simulink model "computed_torque"  (Simulink 8.8)
settings: Solver=FixedStepDiscrete  StartTime=0.0  StopTime=inf  FixedStep=0.01  RelTol=1e-3
InitFcn:
  | WBT_modelName = 'computed-torque';
  | WBT_wbiList = 'ROBOT_TORQUE_CONTROL_JOINTS_WITHOUT_PRONOSUP';
  | 
  | setenv('YARP_ROBOT_NAME','icubGazeboSim');
  | 
  | Dofs = 23;
libraries: WBToolboxLibrary x3
settings Model: SuppressorTable=22 serialization::archive 11 0 3 0 0 0 0 0  Creator=makaveli  LastModifiedBy=makaveli
settings DataIOCC: LimitDataPoints=off  SaveFormat=Dataset  SignalLoggingSaveFormat=Dataset
settings OptimizationCC: LifeSpan=auto
settings DebuggingCC: UnderspecifiedInitializationDetection=Simplified  MergeDetectMultiDrivingBlocksExec=error  FcnCallInpInsideContextMsg=error  StateNameClashWarn=none  SFUnexpectedBacktrackingDiag=error  SFNoUnconditionalDefaultTransitionDiag=error  SFExecutionAtInitializationDiag=warning
settings HardwareCC: ProdBitPerPointer=64  ProdBitPerSizeT=64  ProdBitPerPtrDiffT=64  ProdLargestAtomicFloat=Float  ProdIntDivRoundTo=Zero  ProdEndianess=LittleEndian  ProdWordSize=64  ProdHWDeviceType=Intel->x86-64 (Windows64)
settings ModelReferenceCC: PropagateSignalLabelsOutOfModel=on
settings GRTTargetCC: TargetLangStandard=C99 (ISO)  GeneratePreprocessorConditionals=Use local settings  CombineOutputUpdateFcns=on  GRTInterface=off
settings ConfigComp: CovMetricSettings=dwe  CovHtmlReporting=off  CovSaveCumulativeToWorkspaceVar=off  CovSaveSingleToWorkspaceVar=off  CovExternalEMLEnable=on

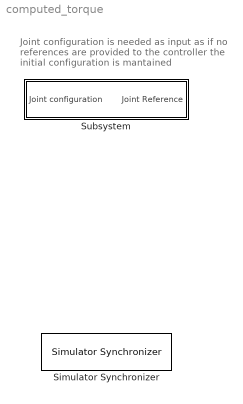
== system computed_torque ==
  note: Joint configuration is needed as input as
      | if no references are provided to the controller
      | the initial configuration is mantained
  Simulator Synchronizer : WBToolboxLibrary/Utilities/Simulator Synchronizer  period=0.01  serverPortName='/clock/rpc'  clientPortName='/WBT_synchronizer/rpc:o'
  Subsystem : Subsystem

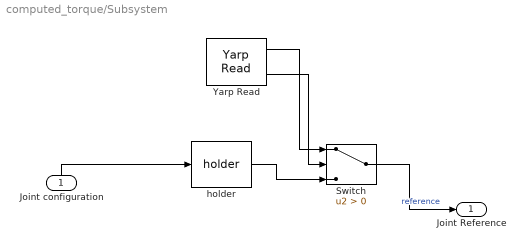
== system computed_torque/Subsystem ==
  Joint configuration : Inport
  Switch : Switch  Criteria=u2 > Threshold
  Yarp Read : WBToolboxLibrary/Utilities/Yarp Read  portName='/computed-torque/qDes:i'  signalSize=Dofs  blocking=off  timestamp=off  autoconnect=off  errorOnConnection=on
  "holder " : WBToolboxLibrary/Utilities/holder 
  Joint Reference : Outport
  wires:
  Switch/1 -> Joint Reference/1  "reference"
  "holder "/1 -> Switch/3
  Yarp Read/2 -> Switch/2
  Yarp Read/1 -> Switch/1
  Joint configuration/1 -> "holder "/1
